simulink library "usask_tlm_lib"  (R2017b)
settings: Solver=ode45  StartTime=0.0  StopTime=10.0  RelTol=1e-3
undefined symbols (not defined in the file or in its folder): B, beta, d, K, L, lambda_1, m_E, m_G, mE_1, mE_2, mG_1, mG_2, nu, r1, r2, rho, T, Zc, Zc_1, Zc_2
libraries: usask_tlm_lib x6, transmission_lines x2
(part 1 of 4)
settings Model: Creator=tkw954  LastModifiedBy=tkw954
settings DataIOCC: LimitDataPoints=on  SaveFormat=Array  SignalLoggingSaveFormat=ModelDataLogs
settings OptimizationCC: BlockReduction=off  BooleanDataType=off  LifeSpan=inf
settings DebuggingCC: SaveWithParameterizedLinksMsg=none  UnderspecifiedInitializationDetection=Classic  MergeDetectMultiDrivingBlocksExec=none  SignalResolutionControl=TryResolveAllWithWarning  MultiTaskDSMMsg=warning  MultiTaskCondExecSysMsg=none  StateNameClashWarn=warning  StrictBusMsg=None  SFUnexpectedBacktrackingDiag=warning  SFNoUnconditionalDefaultTransitionDiag=warning  SFExecutionAtInitializationDiag=none
settings HardwareCC: ProdBitPerPointer=32  ProdBitPerSizeT=32  ProdBitPerPtrDiffT=32  ProdLargestAtomicFloat=None  ProdIntDivRoundTo=Undefined  ProdEndianess=Unspecified  ProdWordSize=32  ProdHWDeviceType=32-bit Generic  TargetUnknown=on
settings ModelReferenceCC: PropagateSignalLabelsOutOfModel=off
settings CodeAppCC: StateflowObjectComments=on
settings GRTTargetCC: TargetLangStandard=C89/C90 (ANSI)  GeneratePreprocessorConditionals=Disable all
settings ConfigComp: CovMetricSettings=dw  CovHtmlReporting=on  CovSaveCumulativeToWorkspaceVar=on  CovSaveSingleToWorkspaceVar=on  CovExternalEMLEnable=off

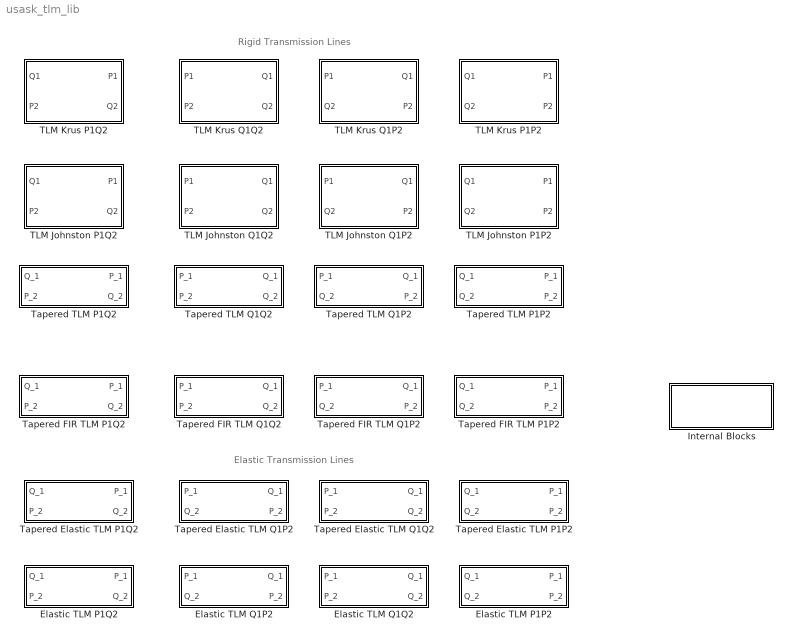
== system usask_tlm_lib ==
  note: Elastic Transmission Lines
  note: Rigid Transmission Lines
  Elastic TLM P1P2 : Subsystem  mask(Elastic Hydraulic Transmission Line (TLM)){K=1.5e9, nu=100e-6, rho=890, D=42e-3, L=10, e_pipe=6e-3, E=190e9, nu_p=0.3, axial_effect=Anchored throughout}
      mask prompts: K "Bulk Modulus (Pa)"; nu "Viscosity (m^2/s)"; rho "Density (kg/m^3)"; D "Diameter (m)"; L "Length (m)"; e_pipe "Wall Thickness (m)"; E "Young's Modulus (Elastic) (Pa)"; nu_p "Poisson's Ratio"; axial_effect "Axial Effect"
      mask help:
      | This model implements the transmission line model in Johnston et al. (2014) with the modifications to include elastic wall effects described in Ghidaoui et al. (2005).
      |
      | This model assumes an elastic tube with a constant wall thickness and a constant radius between the two ports. It assumes constant bulk modulus (no cavitation or entrined air effects) and includes frequency-dependent friction effects.
      |
      | Positive flows are directed into either port. This model also assumes zero initial conditions.
      |
      | "p" is fluid pressure in pascals (Pa).
      | "q" is fluid flow in cubic meters per second (m^3/s).
      | "_1" indicates the inlet, and "_2" indicates the outlet.
      |
      | Reference:
      | N Johnston, M Pan, and S Kudzma. An enhanced transmission line method for modelling laminar flow of liquid in pipelines. Journal of Systems and Control Engineering, 228(4):193–206, 2014.
      |
      | M Ghidaoui, M Zhao, D McInnis, D Axworthy. A Review of Water Hammer Theory and Practice. Transactions of the ASME Applied Mechanics Reviews, Vol 58: 49-76, 2005.
      mask init:
      | %% Note: Equation numbers from:
      | % J ven der Buhs and T Wiens. Modelling Dynamic Response of Hydraulic Fluid Within Tapered 
      | % Transmission Lines. Proceedings of the 15th Scandinavian International Conference on Fluid 
      | % Power, Linköping University, Sweden, 2017.
      | %%
      | 
      | % Check for positive params, report error if negative given
      | if D<0 | L<0 | K<0 | nu<0 | rho<0 | E<0 | e_pipe<0 | nu_p<0
      |     error('Please ensure parameters are all positive')
      | end
      | 
      | r = D/2; % Inlet radius (m)
      | 
      | % Axial effects due to Poisson's ratio (3 models) (Assumes inertial and acceleration effects
      | % of pipe negligable)
      | % 1 = Anchored upstream end only
      | % 2 = Anchored throughout to prevent axial movement
      | % 3 = Pipe with expansion joints throughout
      | % From: Ghidaoui et al. (2005)
      | if axial_effect == 1
      |     alpha = 1 - (nu_p/2);
      | elseif axial_effect == 2;
      |     alpha = 1 - nu_p^2;
      | else
      |     alpha = 1;
      | end
      | 
      | c=sqrt((K./rho)./(1+alpha.*(K./E).*(2.*r./e_pipe)));% Local speed of sound (m/s)
      | beta = (nu.*L)./(c.*r.^2); % Dissipation number (dimensionless), Equation (13)
      | Z_c = (c*rho)/(pi*r^2); % Characteristic impedance (Pa•s/m^3), Equation (10)
      | T=L/c; % Wave propagation time (s)
      | 
      | k=6; % Number of weighting factors
      | 
      | % Grab optimized weighting factors and parameters. Please see paper for
      | % more detail on how these parameters were found.
      | % Parameters are from Johnston et al. (2014)
      | [ni, k2, m_G, m_E, tau] = gettlmcoeffs(beta, k);
      | 
      | if isnan(m_E(1)) | isnan(m_G(1)) | isnan(tau)
      |     error('The parameters you have entered are outside the working range of this model. Weighting factors cannot be found')
      | end  
      |     
      | T_prime = tau*T; % Modified wave propagation time (s), Equation (18) 
      | 
      | n=nan(1,k); % Weighting factor initialization
      | n(1)=0.3/(1+3*beta); % Equation (19)
      | for i=2:k
      |     n(i)=n(i-1)*3; % Equation (19)
      | end
      | 
      | b=1-8*beta/sum(m_E./n); % Equation (16)
      | 
      | %% End of initialization
      mask TypeOptions axial_effect: Anchored inlet | Anchored throughout | Expansion joints throughout
      mask DialogControl DescGroupVar Prompt: Elastic Hydraulic Transmission Line (TLM)
      mask DialogControl Container8 Prompt: Fluid Properties
      mask DialogControl Container8_copy Prompt: Pipeline Parameters
      mask Display:
      | port_label('input', 1 , '\itq_1', 'texmode', 'on')
      | port_label('input', 2 , '\itq_2', 'texmode', 'on')
      | port_label('output', 1 , '\itp_1', 'texmode', 'on')
      | port_label('output', 2 , '\itp_2', 'texmode', 'on')
  Elastic TLM P1Q2 : Subsystem  mask(Elastic Hydraulic Transmission Line (TLM)){K=1.5e9, nu=100e-6, rho=890, D=42e-3, L=10, e_pipe=6e-3, E=190e9, nu_p=0.3, axial_effect=Anchored throughout}
      mask prompts: K "Bulk Modulus (Pa)"; nu "Viscosity (m^2/s)"; rho "Density (kg/m^3)"; D "Diameter (m)"; L "Length (m)"; e_pipe "Wall Thickness (m)"; E "Young's Modulus (Elastic) (Pa)"; nu_p "Poisson's Ratio"; axial_effect "Axial Effect"
      mask help:
      | This model implements the transmission line model in Johnston et al. (2014) with the modifications to include elastic wall effects described in Ghidaoui et al. (2005).
      |
      | This model assumes an elastic tube with a constant wall thickness and a constant radius between the two ports. It assumes constant bulk modulus (no cavitation or entrined air effects) and includes frequency-dependent friction effects.
      |
      | Positive flows are directed into either port. This model also assumes zero initial conditions.
      |
      | "p" is fluid pressure in pascals (Pa).
      | "q" is fluid flow in cubic meters per second (m^3/s).
      | "_1" indicates the inlet, and "_2" indicates the outlet.
      |
      | Reference:
      | N Johnston, M Pan, and S Kudzma. An enhanced transmission line method for modelling laminar flow of liquid in pipelines. Journal of Systems and Control Engineering, 228(4):193–206, 2014.
      |
      | M Ghidaoui, M Zhao, D McInnis, D Axworthy. A Review of Water Hammer Theory and Practice. Transactions of the ASME Applied Mechanics Reviews, Vol 58: 49-76, 2005.
      mask init: same as usask_tlm_lib/Elastic TLM P1P2
      mask TypeOptions axial_effect: Anchored inlet | Anchored throughout | Expansion joints throughout
      mask DialogControl DescGroupVar Prompt: Elastic Hydraulic Transmission Line (TLM)
      mask DialogControl Container8 Prompt: Fluid Properties
      mask DialogControl Container8_copy Prompt: Pipeline Parameters
      mask Display:
      | port_label('input', 1 , '\itq_1', 'texmode', 'on')
      | port_label('input', 2 , '\itp_2', 'texmode', 'on')
      | port_label('output', 1 , '\itp_1', 'texmode', 'on')
      | port_label('output', 2 , '\itq_2', 'texmode', 'on')
  Elastic TLM Q1P2 : Subsystem  mask(Elastic Hydraulic Transmission Line (TLM)){K=1.5e9, nu=100e-6, rho=890, D=42e-3, L=10, e_pipe=6e-3, E=190e9, nu_p=0.3, axial_effect=Anchored throughout}
      mask prompts: K "Bulk Modulus (Pa)"; nu "Viscosity (m^2/s)"; rho "Density (kg/m^3)"; D "Diameter (m)"; L "Length (m)"; e_pipe "Wall Thickness (m)"; E "Young's Modulus (Elastic) (Pa)"; nu_p "Poisson's Ratio"; axial_effect "Axial Effect"
      mask help:
      | This model implements the transmission line model in Johnston et al. (2014) with the modifications to include elastic wall effects described in Ghidaoui et al. (2005).
      |
      | This model assumes an elastic tube with a constant wall thickness and a constant radius between the two ports. It assumes constant bulk modulus (no cavitation or entrined air effects) and includes frequency-dependent friction effects.
      |
      | Positive flows are directed into either port. This model also assumes zero initial conditions.
      |
      | "p" is fluid pressure in pascals (Pa).
      | "q" is fluid flow in cubic meters per second (m^3/s).
      | "_1" indicates the inlet, and "_2" indicates the outlet.
      |
      | Reference:
      | N Johnston, M Pan, and S Kudzma. An enhanced transmission line method for modelling laminar flow of liquid in pipelines. Journal of Systems and Control Engineering, 228(4):193–206, 2014.
      |
      | M Ghidaoui, M Zhao, D McInnis, D Axworthy. A Review of Water Hammer Theory and Practice. Transactions of the ASME Applied Mechanics Reviews, Vol 58: 49-76, 2005.
      mask init: same as usask_tlm_lib/Elastic TLM P1P2
      mask TypeOptions axial_effect: Anchored inlet | Anchored throughout | Expansion joints throughout
      mask DialogControl DescGroupVar Prompt: Elastic Hydraulic Transmission Line (TLM)
      mask DialogControl Container8 Prompt: Fluid Properties
      mask DialogControl Container8_copy Prompt: Pipeline Parameters
      mask Display:
      | port_label('input', 1 , '\itp_1', 'texmode', 'on')
      | port_label('input', 2 , '\itq_2', 'texmode', 'on')
      | port_label('output', 1 , '\itq_1', 'texmode', 'on')
      | port_label('output', 2 , '\itp_2', 'texmode', 'on')
  Elastic TLM Q1Q2 : Subsystem  mask(Elastic Hydraulic Transmission Line (TLM)){K=1.5e9, nu=100e-6, rho=890, D=42e-3, L=10, e_pipe=6e-3, E=190e9, nu_p=0.3, axial_effect=Anchored throughout}
      mask prompts: K "Bulk Modulus (Pa)"; nu "Viscosity (m^2/s)"; rho "Density (kg/m^3)"; D "Diameter (m)"; L "Length (m)"; e_pipe "Wall Thickness (m)"; E "Young's Modulus (Elastic) (Pa)"; nu_p "Poisson's Ratio"; axial_effect "Axial Effect"
      mask help:
      | This model implements the transmission line model in Johnston et al. (2014) with the modifications to include elastic wall effects described in Ghidaoui et al. (2005).
      |
      | This model assumes an elastic tube with a constant wall thickness and a constant radius between the two ports. It assumes constant bulk modulus (no cavitation or entrined air effects) and includes frequency-dependent friction effects.
      |
      | Positive flows are directed into either port. This model also assumes zero initial conditions.
      |
      | "p" is fluid pressure in pascals (Pa).
      | "q" is fluid flow in cubic meters per second (m^3/s).
      | "_1" indicates the inlet, and "_2" indicates the outlet.
      |
      | Reference:
      | N Johnston, M Pan, and S Kudzma. An enhanced transmission line method for modelling laminar flow of liquid in pipelines. Journal of Systems and Control Engineering, 228(4):193–206, 2014.
      |
      | M Ghidaoui, M Zhao, D McInnis, D Axworthy. A Review of Water Hammer Theory and Practice. Transactions of the ASME Applied Mechanics Reviews, Vol 58: 49-76, 2005.
      mask init: same as usask_tlm_lib/Elastic TLM P1P2
      mask TypeOptions axial_effect: Anchored inlet | Anchored throughout | Expansion joints throughout
      mask DialogControl DescGroupVar Prompt: Elastic Hydraulic Transmission Line (TLM)
      mask DialogControl Container8 Prompt: Fluid Properties
      mask DialogControl Container8_copy Prompt: Pipeline Parameters
      mask Display:
      | port_label('input', 1 , '\itp_1', 'texmode', 'on')
      | port_label('input', 2 , '\itp_2', 'texmode', 'on')
      | port_label('output', 1 , '\itq_1', 'texmode', 'on')
      | port_label('output', 2 , '\itq_2', 'texmode', 'on')
  Internal Blocks : Subsystem
  TLM Johnston P1P2 : Subsystem  mask(Transmission Line){L=L, d=d, rho=rho, nu=nu, B=B, modelNumber=2, useCorrected=on}
      mask prompts: L "Length (m)"; d "Diameter (m)"; rho "Density (kg/m^3)"; nu "Kinematic viscosity (m^2/s)"; B "Bulk Modulus (Pa)"; modelNumber "Model Number"; useCorrected "Use corrected impedence"
      mask help:
      | Calculates pipeline dynamics using the Transmission Line Method (TLM).
      |
      | This implementation follows Johnston (2012), which includes an approximation of unsteady laminar flow and frequency-dependent velocity profile. It neglects thermal effects and assumes zero initial pressure and flow.
      |
      | Three models are implemented. Model 1 may be unstable for high beta (see paper). Model 2 is recommended.
      |
      | One may choose to use a more complicated impedence model to compensate for errors in capacitance.
      |
      | Positive flows are into both ports.
      |
      | Reference
      | Johnston, Nigel. "The transmission line method for modelling laminar flow of liquid in pipelines." Proceedings of the Institution of Mechanical Engineers, Part I: Journal of Systems and Control Engineering 226.5 (2012): 586-597.
      mask init:
      | c=sqrt(B/rho);%(m/s) sonic speed
      | 
      | A=pi/4*d^2;%(m^2) cross sectional area
      | r=d/2;%(m) radius
      | T=L/c;%(s) propagation time
      | 
      | R=8*rho*nu*L/(pi*r^4);%(Pa/(m^3/s)) Resistance
      | 
      | K=1.25;%empirical constant
      | 
      | beta=nu*T/r^2;%dissipation number
      | fprintf('beta=%f\n',beta);
      | 
      | k=4;%this must match order of G2 diagram
      | m=nan(k,1);
      | m(1)=2.2457;
      | if k>1
      | m(2)=6.8400;
      | end
      | for i=3:k
      |     m(i)=3*m(i-1);
      | end
      | 
      | 
      | n=nan(k,1);
      | n(1)=42.849;
      | for i=2:k
      |     n(i)=9*n(i-1);
      | end
      | 
      | if useCorrected
      |     Zc=rho*c/A*(1+K*(1-exp(-4*beta))+2*sum(m./n)-4*beta);%(Pa/(m^3/s)) impedence
      | else
      |     Zc=rho*c/A;%(Pa/(m^3/s)) impedence
      | end
      mask TypeOptions modelNumber: 1 | 2 | 3
  TLM Johnston P1Q2 : Subsystem  mask(Transmission Line){L=45, d=13e-3, rho=870, nu=1.2402e-04, B=1.5182e9, modelNumber=2, useCorrected=on}
      mask prompts: L "Length (m)"; d "Diameter (m)"; rho "Density (kg/m^3)"; nu "Kinematic viscosity (m^2/s)"; B "Bulk Modulus (Pa)"; modelNumber "Model Number"; useCorrected "Use corrected impedence"
      mask help:
      | Calculates pipeline dynamics using the Transmission Line Method (TLM).
      |
      | This implementation follows Johnston (2012), which includes an approximation of unsteady laminar flow and frequency-dependent velocity profile. It neglects thermal effects and assumes zero initial pressure and flow.
      |
      | Three models are implemented. Model 1 may be unstable for high beta (see paper). Model 2 is recommended.
      |
      | One may choose to use a more complicated impedence model to compensate for errors in capacitance.
      |
      | Positive flows are into both ports.
      |
      | Reference
      | Johnston, Nigel. "The transmission line method for modelling laminar flow of liquid in pipelines." Proceedings of the Institution of Mechanical Engineers, Part I: Journal of Systems and Control Engineering 226.5 (2012): 586-597.
      mask init: same as usask_tlm_lib/TLM Johnston P1P2
      mask TypeOptions modelNumber: 1 | 2 | 3
  TLM Johnston Q1P2 : Subsystem  mask(Transmission Line){L=45, d=13e-3, rho=870, nu=1.2402e-04, B=1.5182e9, modelNumber=2, useCorrected=on}
      mask prompts: L "Length (m)"; d "Diameter (m)"; rho "Density (kg/m^3)"; nu "Kinematic viscosity (m^2/s)"; B "Bulk Modulus (Pa)"; modelNumber "Model Number"; useCorrected "Use corrected impedence"
      mask help:
      | Calculates pipeline dynamics using the Transmission Line Method (TLM).
      |
      | This implementation follows Johnston (2012), which includes an approximation of unsteady laminar flow and frequency-dependent velocity profile. It neglects thermal effects and assumes zero initial pressure and flow.
      |
      | Three models are implemented. Model 1 may be unstable for high beta (see paper). Model 2 is recommended.
      |
      | One may choose to use a more complicated impedence model to compensate for errors in capacitance.
      |
      | Positive flows are into both ports.
      |
      | Reference
      | Johnston, Nigel. "The transmission line method for modelling laminar flow of liquid in pipelines." Proceedings of the Institution of Mechanical Engineers, Part I: Journal of Systems and Control Engineering 226.5 (2012): 586-597.
      mask init: same as usask_tlm_lib/TLM Johnston P1P2
      mask TypeOptions modelNumber: 1 | 2 | 3
  TLM Johnston Q1Q2 : Subsystem  mask(Transmission Line){L=45, d=13e-3, rho=870, nu=1.2402e-04, B=1.5182e9, modelNumber=2, useCorrected=on}
      mask prompts: L "Length (m)"; d "Diameter (m)"; rho "Density (kg/m^3)"; nu "Kinematic viscosity (m^2/s)"; B "Bulk Modulus (Pa)"; modelNumber "Model Number"; useCorrected "Use corrected impedence"
      mask help:
      | Calculates pipeline dynamics using the Transmission Line Method (TLM).
      |
      | This implementation follows Johnston (2012), which includes an approximation of unsteady laminar flow and frequency-dependent velocity profile. It neglects thermal effects and assumes zero initial pressure and flow.
      |
      | Three models are implemented. Model 1 may be unstable for high beta (see paper). Model 2 is recommended.
      |
      | One may choose to use a more complicated impedence model to compensate for errors in capacitance.
      |
      | Positive flows are into both ports.
      |
      | Reference
      | Johnston, Nigel. "The transmission line method for modelling laminar flow of liquid in pipelines." Proceedings of the Institution of Mechanical Engineers, Part I: Journal of Systems and Control Engineering 226.5 (2012): 586-597.
      mask init: same as usask_tlm_lib/TLM Johnston P1P2
      mask TypeOptions modelNumber: 1 | 2 | 3
  TLM Krus P1P2 : Subsystem  mask(Transmission Line){L=45, d=13e-3, rho=870, nu=1.2402e-04, B=1.5182e9}
      mask prompts: L "Length (m)"; d "Diameter (m)"; rho "Density (kg/m^3)"; nu "Kinematic viscosity (m^2/s)"; B "Bulk Modulus (Pa)"
      mask help:
      | Calculates pipeline dynamics using the Transmission Line Method (TLM).
      |
      | This implementation follows Krus et al (1994), which neglects unsteady friciton and uses simple transfer functions for the filters.
      |
      | Reference
      | Krus P, Weddfelt K and Palmberg J-O. Fast pipeline models for simulation of hydraulic systems. J Dyn Syst Measure Control 1994; 116(1): 132–136.
      mask init:
      | c=sqrt(B/rho);%(m/s) sonic speed
      | 
      | A=pi/4*d^2;%(m^2) cross sectional area
      | r=d/2;%(m) radius
      | T=L/c;%(s) propagation time
      | 
      | R=8*rho*nu*L/(pi*r^4);%(Pa/(m^3/s)) Resistance
      | 
      | K=1.25;%empirical constant
      | 
      | Zc=rho*c/A;%(Pa/(m^3/s)) impedence
      | 
      | beta=nu*T/r^2;%dissipation number
      | fprintf('beta=%f\n',beta);
  TLM Krus P1Q2 : Subsystem  mask(Transmission Line){L=45, d=13e-3, rho=870, nu=1.2402e-04, B=1.5182e9}
      mask prompts: L "Length (m)"; d "Diameter (m)"; rho "Density (kg/m^3)"; nu "Kinematic viscosity (m^2/s)"; B "Bulk Modulus (Pa)"
      mask help:
      | Calculates pipeline dynamics using the Transmission Line Method (TLM).
      |
      | This implementation follows Krus et al (1994), which neglects unsteady friciton and uses simple transfer functions for the filters.
      |
      | Reference
      | Krus P, Weddfelt K and Palmberg J-O. Fast pipeline models for simulation of hydraulic systems. J Dyn Syst Measure Control 1994; 116(1): 132–136.
      mask init: same as usask_tlm_lib/TLM Krus P1P2
  TLM Krus Q1P2 : Subsystem  mask(Transmission Line){L=45, d=13e-3, rho=870, nu=1.2402e-04, B=1.5182e9}
      mask prompts: L "Length (m)"; d "Diameter (m)"; rho "Density (kg/m^3)"; nu "Kinematic viscosity (m^2/s)"; B "Bulk Modulus (Pa)"
      mask help:
      | Calculates pipeline dynamics using the Transmission Line Method (TLM).
      |
      | This implementation follows Krus et al (1994), which neglects unsteady friciton and uses simple transfer functions for the filters.
      |
      | Reference
      | Krus P, Weddfelt K and Palmberg J-O. Fast pipeline models for simulation of hydraulic systems. J Dyn Syst Measure Control 1994; 116(1): 132–136.
      mask init: same as usask_tlm_lib/TLM Krus P1P2
  TLM Krus Q1Q2 : Subsystem  mask(Transmission Line){L=45, d=13e-3, rho=870, nu=1.2402e-04, B=1.5182e9}
      mask prompts: L "Length (m)"; d "Diameter (m)"; rho "Density (kg/m^3)"; nu "Kinematic viscosity (m^2/s)"; B "Bulk Modulus (Pa)"
      mask help:
      | Calculates pipeline dynamics using the Transmission Line Method (TLM).
      |
      | This implementation follows Krus et al (1994), which neglects unsteady friciton and uses simple transfer functions for the filters.
      |
      | Reference
      | Krus P, Weddfelt K and Palmberg J-O. Fast pipeline models for simulation of hydraulic systems. J Dyn Syst Measure Control 1994; 116(1): 132–136.
      mask init: same as usask_tlm_lib/TLM Krus P1P2
  Tapered Elastic TLM P1P2 : Subsystem  mask(Tapered Elastic Hydraulic Transmission Line (TLM)){K=1.5e9, nu=100e-6, rho=890, D_1=40e-3, D_2=42e-3, L=10, e_pipe=3e-3, E=2e9, nu_p=0.3, axial_effect=Anchored throughout}
      mask prompts: K "Oil Bulk Modulus (Pa)"; nu "Oil Viscosity (m^2/s)"; rho "Oil Density (kg/m^3)"; D_1 "Inlet Diameter (m)"; D_2 "Outlet Diameter (m)"; L "Length (m)"; e_pipe "Wall Thickness (m)"; E "Young's Modulus (Elastic) (Pa)"; nu_p "Poisson's Ratio"; axial_effect "Axial Effect"
      mask help:
      | This model implements the transmission line model in ven der Buhs and Wiens (2017). The method uses the the transfer function form from Johnston et. al (2014), however the weighting factors are determined from an optimization procedure comparing to the exact transmission matrix for a tapered pipeline. This model has modifications to include elastic wall effects described in Ghidaoui et al. (2005).
      |
      | This model assumes an elastic tube with a constant wall thickness and a linear taper in radius between the two ports. It assumes constant bulk modulus (no cavitation or entrined air effects) and includes frequency-dependent friction effects.
      |
      | Positive flows are directed into either port. This model also assumes zero initial conditions.
      |
      | "p" is fluid pressure in pascals (Pa).
      | "q" is fluid flow in cubic meters per second (m^3/s).
      | "_1" indicates the inlet, and "_2" indicates the outlet.
      |
      | References:
      | N Johnston, M Pan, and S Kudzma. An enhanced transmission line method for modelling laminar flow of liquid in pipelines. Journal of Systems and Control Engineering, 228(4):193–206, 2014.
      |
      | J ven der Buhs and T Wiens. Modelling Dynamic Response of Hydraulic Fluid Within Tapered Transmission Lines [Submitted]. ASME Journal of Dynamic Systems, Measurement, and Control, 2017.
      |
      | M Ghidaoui, M Zhao, D McInnis, D Axworthy. A Review of Water Hammer Theory and Practice. Transactions of the ASME Applied Mechanics Reviews, Vol 58: 49-76, 2005.
      mask init:
      | %% Note: Equation numbers from: 
      | % J ven der Buhs and T Wiens. Modelling Dynamic Response of Hydraulic Fluid Within Tapered  
      | % Transmission Lines. Proceedings of the 15th Scandinavian International Conference on Fluid Power, Linköping University, Sweden, 2017. %%  
      | 
      | % Check for positive params, report error if negative given 
      | if D_1<0 | D_2<0 | L<0 | K<0 | nu<0 | rho<0 | E<0 | e_pipe<0 | nu_p<0     
      |     error('Please ensure parameters are all positive') 
      | end
      | 
      | r1 = D_1/2; % Inlet radius (m) 
      | r2 = D_2/2; % Outlet radius (m)  
      | 
      | % Axial effects due to Poisson's ratio (3 models) (Assumes inertial and acceleration effects % of pipe negligable) 
      | % 1 = Anchored upstream end only 
      | % 2 = Anchored throughout to prevent axial movement 
      | % 3 = Pipe with expansion joints throughout 
      | % From: Ghidaoui et al. (2005) 
      | 
      | if axial_effect == 1     
      |     alpha = 1 - (nu_p/2); 
      | elseif axial_effect == 2;     
      |     alpha = 1 - nu_p^2;
      | else
      |     alpha = 1;
      | end
      | 
      | fun = @(x) 1./(sqrt((K./rho)./(1+(alpha.*K./E).*(2.*(r1 + (r2-r1)./L.*x)./e_pipe)))); 
      | c_eff = L./integral(fun,0,L); 
      | 
      | lambda = min(r1,r2)/max(r1,r2); % Taper ratio (dimensionless), Equation (11) 
      | beta = ((nu*L)/(c_eff*max(r1,r2)^2))*((lambda^2+lambda+1)^2/(9*lambda^3)); % Dissipation number (dimensionless), Equation (13) 
      | Z_c = ((3*c_eff*rho)/(pi*max(r1,r2)^2))/(lambda^2+lambda+1); % Characteristic impedance (Pa•s/m^3), Equation (10) 
      | T=L/c_eff; % Wave propagation time (s)  
      | k=6; % Number of weighting factors  
      | % Grab optimized weighting factors and parameters. Please see paper for % more detail on how these parameters were found. 
      | [ m_E, m_G, tau ] = interpolateTLMparams( beta, lambda, k);  
      | 
      | if isnan(m_E(1)) | isnan(m_G(1)) | isnan(tau)     
      |     error('The parameters you have entered are outside the working range of this model. Weighting factors cannot be found') 
      | end
      | 
      | T_prime = tau*T; % Modified wave propagation time (s), Equation (18)   
      | n=nan(1,k); % Weighting factor initialization 
      | n(1)=0.3/(1+3*beta); % Equation (19) 
      | for i=2:k     
      |     n(i)=n(i-1)*3; % Equation (19) 
      | end
      | 
      | b=1-8*beta/sum(m_E./n); % Equation (16)
      | 
      | %Error Checking 
      | load TaperedTLMAcceptableErrorContour.mat 
      | IN = inpolygon(lambda,beta,lambda_poly,beta_poly);
      | 
      | if ~IN     
      |     warning('Dissipaton number (beta) and taper ratio (lambda) combination are outside the recommended range') 
      | end
      | 
      | %% End of initialization
      mask TypeOptions axial_effect: Anchored inlet | Anchored throughout | Expansion joints throughout
      mask DialogControl DescGroupVar Prompt: Tapered Hydraulic Transmission Line (TLM)
      mask DialogControl Container4 Prompt: Fluid Properties
      mask DialogControl Container5 Prompt: Pipeline Parameters
      mask Display:
      | port_label('input', 1 , '\itq_1', 'texmode', 'on')
      | port_label('input', 2 , '\itq_2', 'texmode', 'on')
      | port_label('output', 1 , '\itp_1', 'texmode', 'on')
      | port_label('output', 2 , '\itp_2', 'texmode', 'on')
  Tapered Elastic TLM P1Q2 : Subsystem  mask(Tapered Elastic Hydraulic Transmission Line (TLM)){K=1.5e9, nu=100e-6, rho=890, D_1=40e-3, D_2=42e-3, L=10, e_pipe=3e-3, E=2e9, nu_p=0.3, axial_effect=Anchored throughout}
      mask prompts: K "Oil Bulk Modulus (Pa)"; nu "Oil Viscosity (m^2/s)"; rho "Oil Density (kg/m^3)"; D_1 "Inlet Diameter (m)"; D_2 "Outlet Diameter (m)"; L "Length (m)"; e_pipe "Wall Thickness (m)"; E "Young's Modulus (Elastic) (Pa)"; nu_p "Poisson's Ratio"; axial_effect "Axial Effect"
      mask help:
      | This model implements the transmission line model in ven der Buhs and Wiens (2017). The method uses the the transfer function form from Johnston et. al (2014), however the weighting factors are determined from an optimization procedure comparing to the exact transmission matrix for a tapered pipeline. This model has modifications to include elastic wall effects described in Ghidaoui et al. (2005).
      |
      | This model assumes an elastic tube with a constant wall thickness and a linear taper in radius between the two ports. It assumes constant bulk modulus (no cavitation or entrined air effects) and includes frequency-dependent friction effects.
      |
      | Positive flows are directed into either port. This model also assumes zero initial conditions.
      |
      | "p" is fluid pressure in pascals (Pa).
      | "q" is fluid flow in cubic meters per second (m^3/s).
      | "_1" indicates the inlet, and "_2" indicates the outlet.
      |
      | References:
      | N Johnston, M Pan, and S Kudzma. An enhanced transmission line method for modelling laminar flow of liquid in pipelines. Journal of Systems and Control Engineering, 228(4):193–206, 2014.
      |
      | J ven der Buhs and T Wiens. Modelling Dynamic Response of Hydraulic Fluid Within Tapered Transmission Lines [Submitted]. ASME Journal of Dynamic Systems, Measurement, and Control, 2017.
      |
      | M Ghidaoui, M Zhao, D McInnis, D Axworthy. A Review of Water Hammer Theory and Practice. Transactions of the ASME Applied Mechanics Reviews, Vol 58: 49-76, 2005.
      mask init: same as usask_tlm_lib/Tapered Elastic TLM P1P2
      mask TypeOptions axial_effect: Anchored inlet | Anchored throughout | Expansion joints throughout
      mask DialogControl DescGroupVar Prompt: Tapered Hydraulic Transmission Line (TLM)
      mask DialogControl Container4 Prompt: Fluid Properties
      mask DialogControl Container5 Prompt: Pipeline Parameters
      mask Display:
      | port_label('input', 1 , '\itq_1', 'texmode', 'on')
      | port_label('input', 2 , '\itp_2', 'texmode', 'on')
      | port_label('output', 1 , '\itp_1', 'texmode', 'on')
      | port_label('output', 2 , '\itq_2', 'texmode', 'on')
  Tapered Elastic TLM Q1P2 : Subsystem  mask(Tapered Elastic Hydraulic Transmission Line (TLM)){K=1.5e9, nu=100e-6, rho=890, D_1=40e-3, D_2=42e-3, L=10, e_pipe=3e-3, E=2e9, nu_p=0.3, axial_effect=Anchored throughout}
      mask prompts: K "Oil Bulk Modulus (Pa)"; nu "Oil Viscosity (m^2/s)"; rho "Oil Density (kg/m^3)"; D_1 "Inlet Diameter (m)"; D_2 "Outlet Diameter (m)"; L "Length (m)"; e_pipe "Wall Thickness (m)"; E "Young's Modulus (Elastic) (Pa)"; nu_p "Poisson's Ratio"; axial_effect "Axial Effect"
      mask help:
      | This model implements the transmission line model in ven der Buhs and Wiens (2017). The method uses the the transfer function form from Johnston et. al (2014), however the weighting factors are determined from an optimization procedure comparing to the exact transmission matrix for a tapered pipeline. This model has modifications to include elastic wall effects described in Ghidaoui et al. (2005).
      |
      | This model assumes an elastic tube with a constant wall thickness and a linear taper in radius between the two ports. It assumes constant bulk modulus (no cavitation or entrined air effects) and includes frequency-dependent friction effects.
      |
      | Positive flows are directed into either port. This model also assumes zero initial conditions.
      |
      | "p" is fluid pressure in pascals (Pa).
      | "q" is fluid flow in cubic meters per second (m^3/s).
      | "_1" indicates the inlet, and "_2" indicates the outlet.
      |
      | References:
      | N Johnston, M Pan, and S Kudzma. An enhanced transmission line method for modelling laminar flow of liquid in pipelines. Journal of Systems and Control Engineering, 228(4):193–206, 2014.
      |
      | J ven der Buhs and T Wiens. Modelling Dynamic Response of Hydraulic Fluid Within Tapered Transmission Lines [Submitted]. ASME Journal of Dynamic Systems, Measurement, and Control, 2017.
      |
      | M Ghidaoui, M Zhao, D McInnis, D Axworthy. A Review of Water Hammer Theory and Practice. Transactions of the ASME Applied Mechanics Reviews, Vol 58: 49-76, 2005.
      mask init: same as usask_tlm_lib/Tapered Elastic TLM P1P2
      mask TypeOptions axial_effect: Anchored inlet | Anchored throughout | Expansion joints throughout
      mask DialogControl DescGroupVar Prompt: Tapered Hydraulic Transmission Line (TLM)
      mask DialogControl Container4 Prompt: Fluid Properties
      mask DialogControl Container5 Prompt: Pipeline Parameters
      mask Display:
      | port_label('input', 1 , '\itp_1', 'texmode', 'on')
      | port_label('input', 2 , '\itq_2', 'texmode', 'on')
      | port_label('output', 1 , '\itq_1', 'texmode', 'on')
      | port_label('output', 2 , '\itp_2', 'texmode', 'on')
  Tapered Elastic TLM Q1Q2 : Subsystem  mask(Tapered Elastic Hydraulic Transmission Line (TLM)){K=1.5e9, nu=100e-6, rho=890, D_1=40e-3, D_2=42e-3, L=10, e_pipe=3e-3, E=2e9, nu_p=0.3, axial_effect=Anchored throughout}
      mask prompts: K "Oil Bulk Modulus (Pa)"; nu "Oil Viscosity (m^2/s)"; rho "Oil Density (kg/m^3)"; D_1 "Inlet Diameter (m)"; D_2 "Outlet Diameter (m)"; L "Length (m)"; e_pipe "Wall Thickness (m)"; E "Young's Modulus (Elastic) (Pa)"; nu_p "Poisson's Ratio"; axial_effect "Axial Effect"
      mask help:
      | This model implements the transmission line model in ven der Buhs and Wiens (2017). The method uses the the transfer function form from Johnston et. al (2014), however the weighting factors are determined from an optimization procedure comparing to the exact transmission matrix for a tapered pipeline. This model has modifications to include elastic wall effects described in Ghidaoui et al. (2005).
      |
      | This model assumes an elastic tube with a constant wall thickness and a linear taper in radius between the two ports. It assumes constant bulk modulus (no cavitation or entrined air effects) and includes frequency-dependent friction effects.
      |
      | Positive flows are directed into either port. This model also assumes zero initial conditions.
      |
      | "p" is fluid pressure in pascals (Pa).
      | "q" is fluid flow in cubic meters per second (m^3/s).
      | "_1" indicates the inlet, and "_2" indicates the outlet.
      |
      | References:
      | N Johnston, M Pan, and S Kudzma. An enhanced transmission line method for modelling laminar flow of liquid in pipelines. Journal of Systems and Control Engineering, 228(4):193–206, 2014.
      |
      | J ven der Buhs and T Wiens. Modelling Dynamic Response of Hydraulic Fluid Within Tapered Transmission Lines [Submitted]. ASME Journal of Dynamic Systems, Measurement, and Control, 2017.
      |
      | M Ghidaoui, M Zhao, D McInnis, D Axworthy. A Review of Water Hammer Theory and Practice. Transactions of the ASME Applied Mechanics Reviews, Vol 58: 49-76, 2005.
      mask init:
      | %% Note: Equation numbers from: 
      | % J ven der Buhs and T Wiens. Modelling Dynamic Response of Hydraulic Fluid Within Tapered  
      | % Transmission Lines. Proceedings of the 15th Scandinavian International Conference on Fluid Power, Linköping University, Sweden, 2017. %%  
      | 
      | % Check for positive params, report error if negative given 
      | if D_1<0 | D_2<0 | L<0 | K<0 | nu<0 | rho<0 | E<0 | e_pipe<0 | nu_p<0     
      |     error('Please ensure parameters are all positive') 
      | end
      | 
      | r1 = D_1/2; % Inlet radius (m) 
      | r2 = D_2/2; % Outlet radius (m)  
      | 
      | % Axial effects due to Poisson's ratio (3 models) (Assumes inertial and acceleration effects % of pipe negligable) 
      | % 1 = Anchored upstream end only 
      | % 2 = Anchored throughout to prevent axial movement 
      | % 3 = Pipe with expansion joints throughout 
      | % From: Ghidaoui et al. (2005) 
      | 
      | if axial_effect == 1     
      |     alpha = 1 - (nu_p/2); 
      | elseif axial_effect == 2;     
      |     alpha = 1 - nu_p^2;
      | else
      |     alpha = 1;
      | end
      | 
      | fun = @(x) 1./(sqrt((K./rho)./(1+(alpha.*K./E).*(2.*(r1 + (r2-r1)./L.*x)./e_pipe)))); 
      | c_eff = L./integral(fun,0,L); 
      |   
      | lambda = min(r1,r2)/max(r1,r2); % Taper ratio (dimensionless), Equation (11) 
      | beta = ((nu*L)/(c_eff*max(r1,r2)^2))*((lambda^2+lambda+1)^2/(9*lambda^3)); % Dissipation number (dimensionless), Equation (13) 
      | Z_c = ((3*c_eff*rho)/(pi*max(r1,r2)^2))/(lambda^2+lambda+1); % Characteristic impedance (Pa•s/m^3), Equation (10) 
      | T=L/c_eff; % Wave propagation time (s)  
      | k=6; % Number of weighting factors  
      | % Grab optimized weighting factors and parameters. Please see paper for % more detail on how these parameters were found. 
      | [ m_E, m_G, tau ] = interpolateTLMparams( beta, lambda, k);  
      | 
      | if isnan(m_E(1)) | isnan(m_G(1)) | isnan(tau)     
      |     error('The parameters you have entered are outside the working range of this model. Weighting factors cannot be found') 
      | end
      | 
      | T_prime = tau*T; % Modified wave propagation time (s), Equation (18)   
      | n=nan(1,k); % Weighting factor initialization 
      | n(1)=0.3/(1+3*beta); % Equation (19) 
      | for i=2:k     
      |     n(i)=n(i-1)*3; % Equation (19) 
      | end
      | 
      | b=1-8*beta/sum(m_E./n); % Equation (16)
      | 
      | %Error Checking 
      | load TaperedTLMAcceptableErrorContour.mat 
      | IN = inpolygon(lambda,beta,lambda_poly,beta_poly);
      | 
      | if ~IN     
      |     warning('Dissipaton number (beta) and taper ratio (lambda) combination are outside the recommended range') 
      | end
      | 
      | %% End of initialization
      mask TypeOptions axial_effect: Anchored inlet | Anchored throughout | Expansion joints throughout
      mask DialogControl DescGroupVar Prompt: Tapered Hydraulic Transmission Line (TLM)
      mask DialogControl Container4 Prompt: Fluid Properties
      mask DialogControl Container5 Prompt: Pipeline Parameters
      mask Display:
      | port_label('input', 1 , '\itp_1', 'texmode', 'on')
      | port_label('input', 2 , '\itp_2', 'texmode', 'on')
      | port_label('output', 1 , '\itq_1', 'texmode', 'on')
      | port_label('output', 2 , '\itq_2', 'texmode', 'on')
  Tapered FIR TLM P1P2 : Subsystem  mask(Tapered Hydraulic Transmission Line (TLM)){D_1=r1*2, D_2=r2*2, L=L, K=K, nu=nu, rho=rho}
      mask prompts: D_1 "Inlet Diameter (m)"; D_2 "Outlet Diameter (m)"; L "Length (m)"; K "Oil Bulk Modulus (Pa)"; nu "Oil Viscosity (m^2/s)"; rho "Oil Density (kg/m^3)"
      mask help:
      | This model implements the transmission line model in Wiens and ven der Buhs (2018).
      |
      | This model assumes a rigid-walled tube with a linear taper in radius between the two ports. It assumes constant bulk modulus (no cavitation or entrined air effects) and includes frequency-dependent friction effects.
      |
      | Positive flows are directed into either port.
      |
      | This model also assumes zero initial conditions
      |
      | Reference:
      | Travis Wiens and Jeremy vsn der Buhs. In Improved Transmission Line Model for Dynamic Laminar Flow Through Tapered Tubes. Proceedings of the Bath/ASME Symposium on Fluid Power and Motion Control, Bath, 2018
      mask init:
      | %% Note: Equation numbers from:
      | % J ven der Buhs and T Wiens. Modelling Dynamic Response of Hydraulic Fluid Within Tapered
      | % Transmission Lines. Proceedings of the 15th Scandinavian International Conference on Fluid
      | % Power, Linköping University, Sweden, 2017.
      | %%
      | 
      | % Check for positive params, report error if negative given
      | if D_1<0 || D_2<0 || L<0 || K<0 || nu<0 || rho<0
      |     error('Please ensure parameters are all positive')
      | end
      | 
      | r1 = D_1/2; % Inlet radius (m)
      | r2 = D_2/2; % Outlet radius (m)
      | 
      | c=sqrt(K/rho);% Local speed of sound (m/s)
      | lambda_1 = r2/r1; % Taper ratio (dimensionless), Equation (11)
      | %lambda_2 = r1/r2; % Taper ratio (dimensionless), Equation (11)
      | beta = ((nu*L)/(c*r1^2))*((lambda_1^2+lambda_1+1)^2/(9*lambda_1^3)); % Dissipation number (dimensionless), Equation (13)
      | %Z_c = ((3*c*rho)/(pi*max(r1,r2)^2))/(lambda_1^2+lambda_1+1); % Characteristic impedance (Pa•s/m^3), Equation (10)
      | Zc_1=c*rho/(pi*r1^2);
      | Zc_2=c*rho/(pi*r2^2);
      | T=L/c; % Wave propagation time (s)
      | % 
      | % R=Zc_1*beta*8*(3/(1+lambda_1+lambda_1^2));%laminar resistance
      | % 
      | % k=6; % Number of weighting factors
      | % 
      | % % Grab optimized weighting factors and parameters. Please see paper for
      | % % more detail on how these parameters were found.
      | % [ mE_1, mG_1, tau_1, K_diff1, K_mean1 ] = interpolateTLMparamsFIR( beta, lambda_1, k);
      | % [ mE_2, mG_2, tau_2, K_diff2, K_mean2 ] = interpolateTLMparamsFIR( beta, lambda_2, k);
      | % 
      | % %Todo: fix error checkings
      | % % if isnan(mE_1(1)) || isnan(mG_1(1)) || isnan(tau_1)
      | % %     error('The parameters you have entered are outside the working range of this model. Weighting factors cannot be found')
      | % % end
      | % 
      | % T_1 = tau_1*T; % Modified wave propagation time (s), Equation (18)
      | % T_2 = tau_2*T; % Modified wave propagation time (s), Equation (18)
      | % 
      | % n=nan(1,k); % Weighting factor initialization
      | % n(1)=0.3/(1+3*beta); % Equation (19)
      | % for i=2:k
      | %     n(i)=n(i-1)*3; % Equation (19)
      | % end
      | % 
      | % H_1DC=K_mean1*(1/lambda_1.^2 -1)/(8*beta*3/(1+lambda_1+lambda_1^2)+1/lambda_1^2+1);
      | % H_2DC=K_mean2*(1/lambda_2.^2 -1)/(8*beta*3/(1+lambda_2+lambda_2^2)+1/lambda_2^2+1);
      | % 
      | % C_1mean=H_1DC/(2*T_1);
      | % C_2mean=H_2DC/(2*T_2);
      | % 
      | % C_1mean=H_1DC;
      | % C_2mean=H_2DC;
      | % 
      | % C_1a=K_diff1*C_1mean;
      | % C_1b=(2-K_diff1)*C_1mean;
      | % 
      | % C_2a=K_diff2*C_2mean;
      | % C_2b=(2-K_diff2)*C_2mean;
      | % 
      | % 
      | % N_H=100;%make this a parameter
      | % % H_1=[0 linspace(C_1a,C_1b,N_H-1)]./(N_H-1);
      | % % H_2=[0 linspace(C_2a,C_2b,N_H-1)]./(N_H-1);
      | % 
      | % H_1=[linspace(C_1a,C_1b,N_H)]./(N_H);
      | % H_2=[linspace(C_2a,C_2b,N_H)]./(N_H);
      | % 
      | % assignin('base','H_1',H_1);
      | % 
      | % E_1DC=Zc_1*sum(mE_1./n);
      | % E_2DC=Zc_2*sum(mE_2./n);
      | % 
      | % b_1=1-8*beta/(E_1DC/Zc_1);% eq (16)
      | % b_2=1-8*beta/(E_2DC/Zc_2);% eq (16)
      | % 
      | % F_1DC=Zc_1+b_1*E_1DC;
      | % F_2DC=Zc_2+b_2*E_2DC;
      | % 
      | % 
      | % F_k1=((1-H_1DC)*(E_2DC+Zc_2-R)+H_2DC*(E_1DC+Zc_1))/(1-H_1DC-H_2DC)/F_1DC
      | % F_k2=((1-H_2DC)*(E_1DC+Zc_1-R)+H_1DC*(E_2DC+Zc_2))/(1-H_2DC-H_1DC)/F_2DC
      | % %F_k1=1;
      | % %F_k2=1;
      | % 
      | % %G_DC1=(1-H_DC2);
      | % %G_DC2=(1-H_DC1);
      | % 
      | % %Error Checking
      | % % load TaperedTLMAcceptableErrorContour.mat
      | % % IN = inpolygon(lambda_1,beta,lambda_poly,beta_poly);
      | % % if ~IN
      | % %     warning('Dissipaton number (beta) and taper ratio (lambda) combination are outside the recommended range')
      | % % end
      | % warning('need to reinstate polygon error checking')
      | % 
      | % 
      | % 
      | % 
      | % %% End of initialization
      mask DialogControl DescGroupVar Prompt: Tapered Hydraulic Transmission Line (TLM)
      mask Display:
      | port_label('input', 1 , '\itq_1', 'texmode', 'on')
      | port_label('input', 2 , '\itq_2', 'texmode', 'on')
      | port_label('output', 1 , '\itp_1', 'texmode', 'on')
      | port_label('output', 2 , '\itp_2', 'texmode', 'on')
  Tapered FIR TLM P1Q2 : Subsystem  mask(Tapered Hydraulic Transmission Line (TLM)){D_1=r1*2, D_2=r2*2, L=L, K=K, nu=nu, rho=rho}
      mask prompts: D_1 "Inlet Diameter (m)"; D_2 "Outlet Diameter (m)"; L "Length (m)"; K "Oil Bulk Modulus (Pa)"; nu "Oil Viscosity (m^2/s)"; rho "Oil Density (kg/m^3)"
      mask help:
      | This model implements the transmission line model in Wiens and ven der Buhs (2018).
      |
      | This model assumes a rigid-walled tube with a linear taper in radius between the two ports. It assumes constant bulk modulus (no cavitation or entrined air effects) and includes frequency-dependent friction effects.
      |
      | Positive flows are directed into either port.
      |
      | This model also assumes zero initial conditions
      |
      | Reference:
      | Travis Wiens and Jeremy vsn der Buhs. In Improved Transmission Line Model for Dynamic Laminar Flow Through Tapered Tubes. Proceedings of the Bath/ASME Symposium on Fluid Power and Motion Control, Bath, 2018
      mask init: same as usask_tlm_lib/Tapered FIR TLM P1P2
      mask DialogControl DescGroupVar Prompt: Tapered Hydraulic Transmission Line (TLM)
      mask Display:
      | port_label('input', 1 , '\itq_1', 'texmode', 'on')
      | port_label('input', 2 , '\itp_2', 'texmode', 'on')
      | port_label('output', 1 , '\itp_1', 'texmode', 'on')
      | port_label('output', 2 , '\itq_2', 'texmode', 'on')
  Tapered FIR TLM Q1P2 : Subsystem  mask(Tapered Hydraulic Transmission Line (TLM)){D_1=10e-3, D_2=15e-3, L=10, K=1e9, nu=60e-6, rho=890}
      mask prompts: D_1 "Inlet Diameter (m)"; D_2 "Outlet Diameter (m)"; L "Length (m)"; K "Oil Bulk Modulus (Pa)"; nu "Oil Viscosity (m^2/s)"; rho "Oil Density (kg/m^3)"
      mask help:
      | This model implements the transmission line model in Wiens and ven der Buhs (2018).
      |
      | This model assumes a rigid-walled tube with a linear taper in radius between the two ports. It assumes constant bulk modulus (no cavitation or entrined air effects) and includes frequency-dependent friction effects.
      |
      | Positive flows are directed into either port.
      |
      | This model also assumes zero initial conditions
      |
      | Reference:
      | Travis Wiens and Jeremy vsn der Buhs. In Improved Transmission Line Model for Dynamic Laminar Flow Through Tapered Tubes. Proceedings of the Bath/ASME Symposium on Fluid Power and Motion Control, Bath, 2018
      mask init: same as usask_tlm_lib/Tapered FIR TLM P1P2
      mask DialogControl DescGroupVar Prompt: Tapered Hydraulic Transmission Line (TLM)
      mask Display:
      | port_label('input', 1 , '\itp_1', 'texmode', 'on')
      | port_label('input', 2 , '\itq_2', 'texmode', 'on')
      | port_label('output', 1 , '\itq_1', 'texmode', 'on')
      | port_label('output', 2 , '\itp_2', 'texmode', 'on')
  Tapered FIR TLM Q1Q2 : Subsystem  mask(Tapered Hydraulic Transmission Line (TLM)){D_1=r1*2, D_2=r2*2, L=L, K=K, nu=nu, rho=rho}
      mask prompts: D_1 "Inlet Diameter (m)"; D_2 "Outlet Diameter (m)"; L "Length (m)"; K "Oil Bulk Modulus (Pa)"; nu "Oil Viscosity (m^2/s)"; rho "Oil Density (kg/m^3)"
      mask help:
      | This model implements the transmission line model in Wiens and ven der Buhs (2018).
      |
      | This model assumes a rigid-walled tube with a linear taper in radius between the two ports. It assumes constant bulk modulus (no cavitation or entrined air effects) and includes frequency-dependent friction effects.
      |
      | Positive flows are directed into either port.
      |
      | This model also assumes zero initial conditions
      |
      | Reference:
      | Travis Wiens and Jeremy vsn der Buhs. In Improved Transmission Line Model for Dynamic Laminar Flow Through Tapered Tubes. Proceedings of the Bath/ASME Symposium on Fluid Power and Motion Control, Bath, 2018
      mask init: same as usask_tlm_lib/Tapered FIR TLM P1P2
      mask DialogControl DescGroupVar Prompt: Tapered Hydraulic Transmission Line (TLM)
      mask Display:
      | port_label('input', 1 , '\itp_1', 'texmode', 'on')
      | port_label('input', 2 , '\itp_2', 'texmode', 'on')
      | port_label('output', 1 , '\itq_1', 'texmode', 'on')
      | port_label('output', 2 , '\itq_2', 'texmode', 'on')
  Tapered TLM P1P2 : Subsystem  mask(Tapered Hydraulic Transmission Line (TLM)){D_1=40e-3, D_2=42e-3, L=10, K=1.5e9, nu=100e-6, rho=890}
      mask prompts: D_1 "Inlet Diameter (m)"; D_2 "Outlet Diameter (m)"; L "Length (m)"; K "Oil Bulk Modulus (Pa)"; nu "Oil Viscosity (m^2/s)"; rho "Oil Density (kg/m^3)"
      mask help:
      | This model implements the transmission line model in ven der Buhs and Wiens (2017). The method uses the the transfer function form from Johnston et. al (2014), however the weighting factors are determined from an optimization procedure comparing to the exact transmission matrix for a tapered pipeline.
      |
      | This model assumes a rigid-walled tube with a linear taper in radius between the two ports. It assumes constant bulk modulus (no cavitation or entrined air effects) and includes frequency-dependent friction effects.
      |
      | Positive flows are directed into either port.
      |
      | This model also assumes zero initial conditions
      |
      | Reference:
      | N Johnston, M Pan, and S Kudzma. An enhanced transmission line method for modelling laminar flow of liquid in pipelines. Journal of Systems and Control Engineering, 228(4):193–206, 2014.
      |
      | J ven der Buhs and T Wiens. Modelling Dynamic Response of Hydraulic Fluid Within Tapered Transmission Lines. Proceedings of the 15th Scandinavian International Conference on Fluid Power, 2017
      mask init:
      | %% Note: Equation numbers from:
      | % J ven der Buhs and T Wiens. Modelling Dynamic Response of Hydraulic Fluid Within Tapered 
      | % Transmission Lines. Proceedings of the 15th Scandinavian International Conference on Fluid 
      | % Power, Linköping University, Sweden, 2017.
      | %%
      | 
      | % Check for positive params, report error if negative given
      | if D_1<0 | D_2<0 | L<0 | K<0 | nu<0 | rho<0
      |     error('Please ensure parameters are all positive')
      | end
      | 
      | r1 = D_1/2; % Inlet radius (m)
      | r2 = D_2/2; % Outlet radius (m)
      | 
      | c=sqrt(K/rho);% Local speed of sound (m/s)
      | lambda = min(r1,r2)/max(r1,r2); % Taper ratio (dimensionless), Equation (11)
      | beta = ((nu*L)/(c*max(r1,r2)^2))*((lambda^2+lambda+1)^2/(9*lambda^3)); % Dissipation number (dimensionless), Equation (13)
      | Z_c = ((3*c*rho)/(pi*max(r1,r2)^2))/(lambda^2+lambda+1); % Characteristic impedance (Pa•s/m^3), Equation (10)
      | T=L/c; % Wave propagation time (s)
      | 
      | k=6; % Number of weighting factors
      | 
      | % Grab optimized weighting factors and parameters. Please see paper for
      | % more detail on how these parameters were found.
      | [ m_E, m_G, tau ] = interpolateTLMparams( beta, lambda, k);
      | 
      | if isnan(m_E(1)) | isnan(m_G(1)) | isnan(tau)
      |     error('The parameters you have entered are outside the working range of this model. Weighting factors cannot be found')
      | end  
      |     
      | T_prime = tau*T; % Modified wave propagation time (s), Equation (18) 
      | 
      | n=nan(1,k); % Weighting factor initialization
      | n(1)=0.3/(1+3*beta); % Equation (19)
      | for i=2:k
      |     n(i)=n(i-1)*3; % Equation (19)
      | end
      | 
      | b=1-8*beta/sum(m_E./n); % Equation (16)
      | 
      | %Error Checking
      | load TaperedTLMAcceptableErrorContour.mat
      | IN = inpolygon(lambda,beta,lambda_poly,beta_poly);
      | if ~IN
      |     warning('Dissipaton number (beta) and taper ratio (lambda) combination are outside the recommended range')
      | end
      | 
      | 
      | 
      | 
      | %% End of initialization
      mask DialogControl DescGroupVar Prompt: Tapered Hydraulic Transmission Line (TLM)
      mask Display:
      | port_label('input', 1 , '\itq_1', 'texmode', 'on')
      | port_label('input', 2 , '\itq_2', 'texmode', 'on')
      | port_label('output', 1 , '\itp_1', 'texmode', 'on')
      | port_label('output', 2 , '\itp_2', 'texmode', 'on')
  Tapered TLM P1Q2 : Subsystem  mask(Tapered Hydraulic Transmission Line (TLM)){D_1=40e-3, D_2=42e-3, L=10, K=1.5e9, nu=100e-6, rho=890}
      mask prompts: D_1 "Inlet Diameter (m)"; D_2 "Outlet Diameter (m)"; L "Length (m)"; K "Oil Bulk Modulus (Pa)"; nu "Oil Viscosity (m^2/s)"; rho "Oil Density (kg/m^3)"
      mask help:
      | This model implements the transmission line model in ven der Buhs and Wiens (2017). The method uses the the transfer function form from Johnston et. al (2014), however the weighting factors are determined from an optimization procedure comparing to the exact transmission matrix for a tapered pipeline.
      |
      | This model assumes a rigid-walled tube with a linear taper in radius between the two ports. It assumes constant bulk modulus (no cavitation or entrined air effects) and includes frequency-dependent friction effects.
      |
      | Positive flows are directed into either port. This model also assumes zero initial conditions.
      |
      | "p" is fluid pressure in pascals (Pa).
      | "q" is fluid flow in cubic meters per second (m^3/s).
      | "_1" indicates the inlet, and "_2" indicates the outlet.
      |
      | Reference:
      | N Johnston, M Pan, and S Kudzma. An enhanced transmission line method for modelling laminar flow of liquid in pipelines. Journal of Systems and Control Engineering, 228(4):193–206, 2014.
      |
      | J ven der Buhs and T Wiens. Modelling Dynamic Response of Hydraulic Fluid Within Tapered Transmission Lines. Proceedings of the 15th Scandinavian International Conference on Fluid Power, Linköping University, Sweden, 2017.
      mask init: same as usask_tlm_lib/Tapered TLM P1P2
      mask DialogControl DescGroupVar Prompt: Tapered Hydraulic Transmission Line (TLM)
      mask Display:
      | port_label('input', 1 , '\itq_1', 'texmode', 'on')
      | port_label('input', 2 , '\itp_2', 'texmode', 'on')
      | port_label('output', 1 , '\itp_1', 'texmode', 'on')
      | port_label('output', 2 , '\itq_2', 'texmode', 'on')
  Tapered TLM Q1P2 : Subsystem  mask(Tapered Hydraulic Transmission Line (TLM)){D_1=40e-3, D_2=42e-3, L=10, K=1.5e9, nu=100e-6, rho=890}
      mask prompts: D_1 "Inlet Diameter (m)"; D_2 "Outlet Diameter (m)"; L "Length (m)"; K "Oil Bulk Modulus (Pa)"; nu "Oil Viscosity (m^2/s)"; rho "Oil Density (kg/m^3)"
      mask help:
      | This model implements the transmission line model in ven der Buhs and Wiens (2017). The method uses the the transfer function form from Johnston et. al (2014), however the weighting factors are determined from an optimization procedure comparing to the exact transmission matrix for a tapered pipeline.
      |
      | This model assumes a rigid-walled tube with a linear taper in radius between the two ports. It assumes constant bulk modulus (no cavitation or entrined air effects) and includes frequency-dependent friction effects.
      |
      | Positive flows are directed into either port.
      |
      | This model also assumes zero initial conditions
      |
      | Reference:
      | N Johnston, M Pan, and S Kudzma. An enhanced transmission line method for modelling laminar flow of liquid in pipelines. Journal of Systems and Control Engineering, 228(4):193–206, 2014.
      |
      | J ven der Buhs and T Wiens. Modelling Dynamic Response of Hydraulic Fluid Within Tapered Transmission Lines. Proceedings of the 15th Scandinavian International Conference on Fluid Power, 2017
      mask init: same as usask_tlm_lib/Tapered TLM P1P2
      mask DialogControl DescGroupVar Prompt: Tapered Hydraulic Transmission Line (TLM)
      mask Display:
      | port_label('input', 1 , '\itp_1', 'texmode', 'on')
      | port_label('input', 2 , '\itq_2', 'texmode', 'on')
      | port_label('output', 1 , '\itq_1', 'texmode', 'on')
      | port_label('output', 2 , '\itp_2', 'texmode', 'on')
  Tapered TLM Q1Q2 : Subsystem  mask(Tapered Hydraulic Transmission Line (TLM)){D_1=40e-3, D_2=42e-3, L=10, K=1.5e9, nu=100e-6, rho=890}
      mask prompts: D_1 "Inlet Diameter (m)"; D_2 "Outlet Diameter (m)"; L "Length (m)"; K "Oil Bulk Modulus (Pa)"; nu "Oil Viscosity (m^2/s)"; rho "Oil Density (kg/m^3)"
      mask help:
      | This model implements the transmission line model in ven der Buhs and Wiens (2017). The method uses the the transfer function form from Johnston et. al (2014), however the weighting factors are determined from an optimization procedure comparing to the exact transmission matrix for a tapered pipeline.
      |
      | This model assumes a rigid-walled tube with a linear taper in radius between the two ports. It assumes constant bulk modulus (no cavitation or entrined air effects) and includes frequency-dependent friction effects.
      |
      | Positive flows are directed into either port.
      |
      | This model also assumes zero initial conditions
      |
      | Reference:
      | N Johnston, M Pan, and S Kudzma. An enhanced transmission line method for modelling laminar flow of liquid in pipelines. Journal of Systems and Control Engineering, 228(4):193–206, 2014.
      |
      | J ven der Buhs and T Wiens. Modelling Dynamic Response of Hydraulic Fluid Within Tapered Transmission Lines. Proceedings of the 15th Scandinavian International Conference on Fluid Power, 2017
      mask init: same as usask_tlm_lib/Tapered TLM P1P2
      mask DialogControl DescGroupVar Prompt: Tapered Hydraulic Transmission Line (TLM)
      mask Display:
      | port_label('input', 1 , '\itp_1', 'texmode', 'on')
      | port_label('input', 2 , '\itp_2', 'texmode', 'on')
      | port_label('output', 1 , '\itq_1', 'texmode', 'on')
      | port_label('output', 2 , '\itq_2', 'texmode', 'on')
